simulink library "quadLibrary"  (R2015b)
settings: Solver=VariableStepAuto  StartTime=0.0  StopTime=10.0  RelTol=1e-3
settings Model: Creator=Nik Descher  LastModifiedBy=Nik Descher

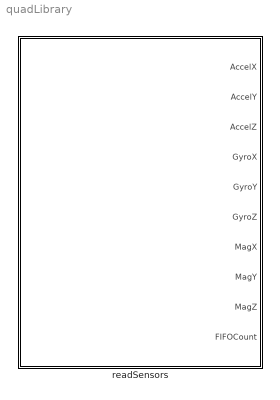
== system quadLibrary ==
  readSensors : Subsystem  TreatAsAtomicUnit=on  SystemSampleTime=1/1000

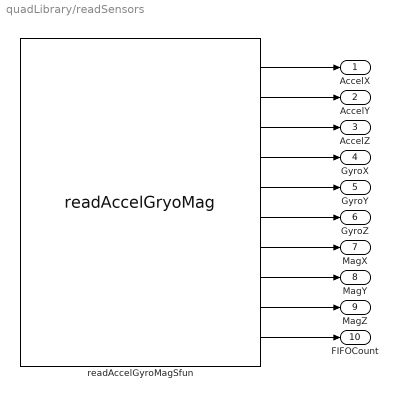
== system quadLibrary/readSensors ==
  readAccelGyroMagSfun : S-Function  InitFcn=try, set_param(gcb,'FunctionName','readAccelGryoMag'), end  FunctionName=readAccelGryoMag  SFunctionModules=readAccelGryoMag_wrapper  SFunctionDeploymentMode=off  EnableBusSupport=off  mask(S-Function Builder){Parameter1=0, Parameter2=0}
      mask prompts: Parameter1 "High Reg Address"; Parameter2 "Low Reg Address"
      mask help: Simulink:masks:SFunctionBuilder_MD
      mask init:
      | val = [[.9  0.75 0.75 1 1 .9 .9 1]',[1 1 0.75 0.75 .9 .9 1 .9]'];try , sys = get_param(gcb,'SfunBuilderFcnName');if isempty(sys), sys = get_param(gcb,'FunctionName'); end,catch, sys = get_param(gcb,'FunctionName'); end
      settings: CopyFcn=set_param(gcbh,'LinkStatus','none')  PreSaveFcn=try, set_param(gcb,'FunctionName','readAccelGryoMag'), end  OpenFcn=sfunctionwizard(gcbh)
      mask Display: plot(val(:,1),val(:,2)),disp(sys), port_label('output',1,'AccelX'), port_label('output',2,'AccelY'), port_label('output',3,'AccelZ'), port_label('output',4,'GyroX'), port_label('output',5,'GyroY'), port_label('output',6,'GyroZ'), port_label('output',7,'MagX'), port_label('output',8,'MagY'), port_label('output',9,'MagZ'), port_label('output',10,'FIFOCount')
  AccelX : Outport
  AccelY : Outport  Port=2
  AccelZ : Outport  Port=3
  GyroX : Outport  Port=4
  GyroY : Outport  Port=5
  GyroZ : Outport  Port=6
  MagX : Outport  Port=7
  MagY : Outport  Port=8
  MagZ : Outport  Port=9
  FIFOCount : Outport  Port=10
  wires:
  readAccelGyroMagSfun/10 -> FIFOCount/1
  readAccelGyroMagSfun/5 -> GyroY/1
  readAccelGyroMagSfun/2 -> AccelY/1
  readAccelGyroMagSfun/1 -> AccelX/1
  readAccelGyroMagSfun/4 -> GyroX/1
  readAccelGyroMagSfun/6 -> GyroZ/1
  readAccelGyroMagSfun/7 -> MagX/1
  readAccelGyroMagSfun/3 -> AccelZ/1
  readAccelGyroMagSfun/9 -> MagZ/1
  readAccelGyroMagSfun/8 -> MagY/1
